simulink model "test"  (R2020a)
settings: Solver=VariableStepAuto  StartTime=0.0  StopTime=10.0  RelTol=1e-3
libraries: simulink x6, robotcorelib x2
settings Model: Creator=javier  LastModifiedBy=javier

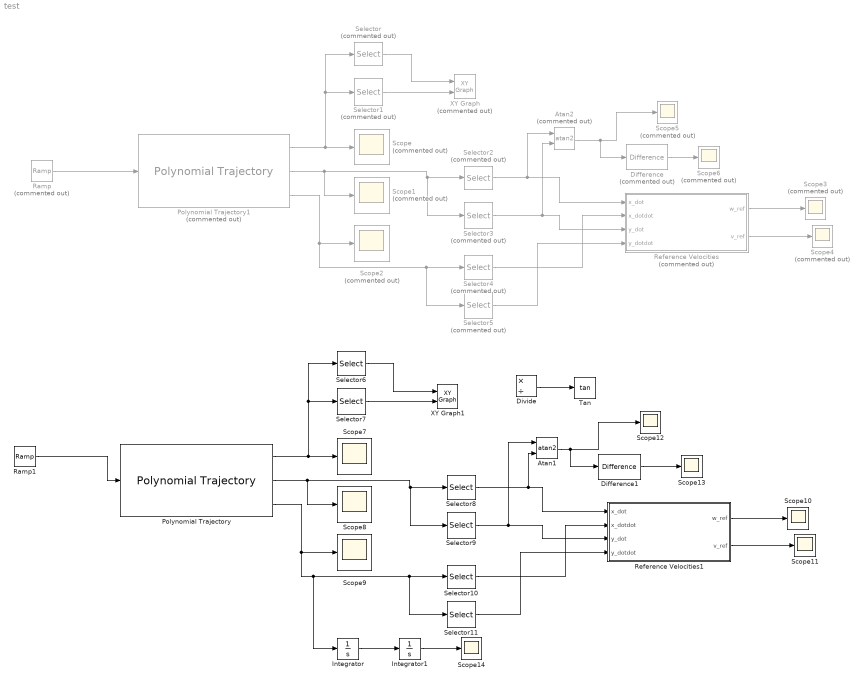
== system test ==
  Atan1 : Trigonometry  Operator=atan2  OutputSignalType=real
  Atan2 : Trigonometry  Commented=on  Operator=atan2
  Difference : simulink/Discrete/Difference  Commented=on  ICPrevInput=0.0  OutMin=[]  OutMax=[]  OutDataType=fixdt(1, 16)  OutScaling=2^-10  DoSatur=off
  Difference1 : simulink/Discrete/Difference  ICPrevInput=0  OutMin=[]  OutMax=[]  OutDataType=fixdt(1, 16)  OutScaling=2^-10  DoSatur=off
  Divide : Product  Inputs=*/
  Integrator : Integrator
  Integrator1 : Integrator
  Polynomial Trajectory : robotcorelib/Polynomial Trajectory  WaypointSource=Internal  Waypoints=[ 0, 0.5, 1, 1.5, 2, 2.5, 3; 0, 0.5, 1, 1, 1, 0.5, 0]  TimePoints=[ 0, 1, 2, 3, 4, 5, 6]  TimeInterval=[ 1, 4]  Method=Cubic Polynomial  ParameterSource=Internal  VelocityBoundaryCondition=zeros( 2, 7 )  AccelerationBoundaryCondition=zeros( 2, 4 )  SimulateUsing=Interpreted execution
      settings: SourceProductBaseCode=NV,RO,RR
  Polynomial Trajectory1 : robotcorelib/Polynomial Trajectory  Commented=on  WaypointSource=Internal  Waypoints=[ 0, 2, 1, 5, 0; -1, 3, 1, 4, 4 ]  TimePoints=[ 0, 1, 2, 3, 4 ]  TimeInterval=[ 1, 4 ]  Method=Cubic Polynomial  ParameterSource=Internal  VelocityBoundaryCondition=zeros( 2, 5 )  AccelerationBoundaryCondition=zeros( 2, 5 )  SimulateUsing=Interpreted execution
      settings: SourceProductBaseCode=NV,RO,RR
  Ramp : simulink/Sources/Ramp  Commented=on  slope=1  start=0  InitialOutput=0
  Ramp1 : simulink/Sources/Ramp  slope=1  start=0  InitialOutput=0
  Reference Velocities : Subsystem  Commented=on
  Reference Velocities1 : Subsystem
  Scope{,1..6} (7 alike) : Scope  Commented=on
  Scope{7..14} (8 alike) : Scope
  Selector : Selector  Commented=on  InputPortWidth=2  IndexOptions=Index vector (dialog)  Indices=1  OutputSizes=1
  Selector1 : Selector  Commented=on  InputPortWidth=2  IndexOptions=Index vector (dialog)  Indices=2  OutputSizes=1
  Selector10 : Selector  InputPortWidth=2  IndexOptions=Index vector (dialog)  Indices=1  OutputSizes=1
  Selector11 : Selector  InputPortWidth=2  IndexOptions=Index vector (dialog)  Indices=2  OutputSizes=1
  Selector2 : Selector  Commented=on  InputPortWidth=2  IndexOptions=Index vector (dialog)  Indices=1  OutputSizes=1
  Selector3 : Selector  Commented=on  InputPortWidth=2  IndexOptions=Index vector (dialog)  Indices=2  OutputSizes=1
  Selector4 : Selector  Commented=on  InputPortWidth=2  IndexOptions=Index vector (dialog)  Indices=1  OutputSizes=1
  Selector5 : Selector  Commented=on  InputPortWidth=2  IndexOptions=Index vector (dialog)  Indices=2  OutputSizes=1
  Selector6 : Selector  InputPortWidth=2  IndexOptions=Index vector (dialog)  Indices=1  OutputSizes=1
  Selector7 : Selector  InputPortWidth=2  IndexOptions=Index vector (dialog)  Indices=2  OutputSizes=1
  Selector8 : Selector  InputPortWidth=2  IndexOptions=Index vector (dialog)  Indices=1  OutputSizes=1
  Selector9 : Selector  InputPortWidth=2  IndexOptions=Index vector (dialog)  Indices=2  OutputSizes=1
  Tan : Trigonometry  Operator=tan
  XY Graph : simulink/Sinks/XY Graph  Commented=on  xmin=-3  xmax=5  ymin=-1  ymax=5  st=-1
  XY Graph1 : simulink/Sinks/XY Graph  xmin=-3  xmax=5  ymin=-1  ymax=5  st=-1
  wires:
  Polynomial Trajectory1/1 -> Selector1/1, Selector/1, Scope/1
  Polynomial Trajectory1/2 -> Selector3/1, Selector2/1, Scope1/1
  Selector3/1 -> Atan2/2, Reference Velocities/3(y_dot)
  Reference Velocities/1(w_ref) -> Scope3/1
  Polynomial Trajectory1/3 -> Scope2/1, Selector5/1, Selector4/1
  Selector4/1 -> Reference Velocities/2(x_dotdot)
  Atan2/1 -> Difference/1, Scope5/1
  Selector/1 -> XY Graph/1
  Selector2/1 -> Atan2/1, Reference Velocities/1(x_dot)
  Ramp/1 -> Polynomial Trajectory1/1
  Reference Velocities/2(v_ref) -> Scope4/1
  Difference/1 -> Scope6/1
  Selector5/1 -> Reference Velocities/4(y_dotdot)
  Selector1/1 -> XY Graph/2
  Selector9/1 -> Atan1/1, Reference Velocities1/3(y_dot)
  Polynomial Trajectory/2 -> Selector9/1, Selector8/1, Scope8/1
  Ramp1/1 -> Polynomial Trajectory/1
  Reference Velocities1/1(w_ref) -> Scope10/1
  Reference Velocities1/2(v_ref) -> Scope11/1
  Selector10/1 -> Reference Velocities1/2(x_dotdot)
  Selector8/1 -> Atan1/2, Reference Velocities1/1(x_dot)
  Polynomial Trajectory/1 -> Selector7/1, Selector6/1, Scope7/1
  Selector11/1 -> Reference Velocities1/4(y_dotdot)
  Polynomial Trajectory/3 -> Scope9/1, Integrator/1, Selector11/1, Selector10/1
  Atan1/1 -> Difference1/1, Scope12/1
  Selector6/1 -> XY Graph1/1
  Selector7/1 -> XY Graph1/2
  Integrator/1 -> Integrator1/1
  Integrator1/1 -> Scope14/1
  Difference1/1 -> Scope13/1
  Divide/1 -> Tan/1

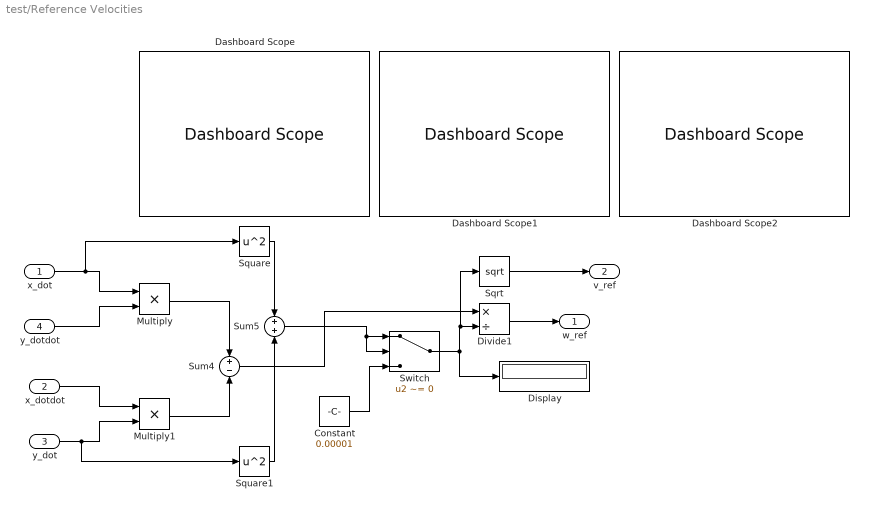
== system test/Reference Velocities ==
  x_dot : Inport
  x_dotdot : Inport  Port=2
  y_dot : Inport  Port=3
  y_dotdot : Inport  Port=4
  Constant : Constant  Value=0.00001
  Dashboard Scope : DashboardScope
  Dashboard Scope1 : DashboardScope
  Dashboard Scope2 : DashboardScope
  Display : Display
  Divide1 : Product  Inputs=*/  OutMin=[0.0000001]
  Multiply : Product
  Multiply1 : Product
  Sqrt : Sqrt  SaturateOnIntegerOverflow=on
  Square : Math  Operator=square  SignedPower=on  SaturateOnIntegerOverflow=on
  Square1 : Math  Operator=square  SignedPower=on  SaturateOnIntegerOverflow=on
  Sum4 : Sum  Inputs=+-
  Sum5 : Sum
  Switch : Switch  Criteria=u2 ~= 0
  w_ref : Outport  VectorParamsAs1DForOutWhenUnconnected=off
  v_ref : Outport  Port=2  VectorParamsAs1DForOutWhenUnconnected=off
  wires:
  x_dot/1 -> Square/1, Multiply/1
  Divide1/1 -> w_ref/1
  x_dotdot/1 -> Multiply1/1
  Square/1 -> Sum5/1
  Sum4/1 -> Divide1/1
  y_dot/1 -> Square1/1, Multiply1/2
  y_dotdot/1 -> Multiply/2
  Multiply1/1 -> Sum4/2
  Square1/1 -> Sum5/2
  Multiply/1 -> Sum4/1
  Sqrt/1 -> v_ref/1
  Constant/1 -> Switch/3
  Sum5/1 -> Switch/2, Switch/1
  Switch/1 -> Display/1, Sqrt/1, Divide1/2

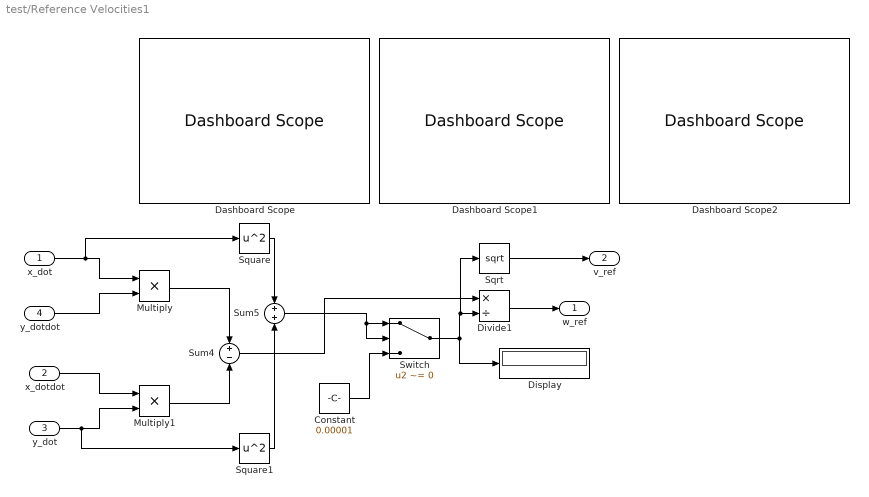
== system test/Reference Velocities1 ==
  x_dot : Inport
  x_dotdot : Inport  Port=2
  y_dot : Inport  Port=3
  y_dotdot : Inport  Port=4
  Constant : Constant  Value=0.00001
  Dashboard Scope : DashboardScope
  Dashboard Scope1 : DashboardScope
  Dashboard Scope2 : DashboardScope
  Display : Display
  Divide1 : Product  Inputs=*/  OutMin=[0.0000001]
  Multiply : Product
  Multiply1 : Product
  Sqrt : Sqrt  SaturateOnIntegerOverflow=on
  Square : Math  Operator=square  SignedPower=on  SaturateOnIntegerOverflow=on
  Square1 : Math  Operator=square  SignedPower=on  SaturateOnIntegerOverflow=on
  Sum4 : Sum  Inputs=+-
  Sum5 : Sum
  Switch : Switch  Criteria=u2 ~= 0
  w_ref : Outport  VectorParamsAs1DForOutWhenUnconnected=off
  v_ref : Outport  Port=2  VectorParamsAs1DForOutWhenUnconnected=off
  wires:
  x_dot/1 -> Square/1, Multiply/1
  Divide1/1 -> w_ref/1
  x_dotdot/1 -> Multiply1/1
  Square/1 -> Sum5/1
  Sum4/1 -> Divide1/1
  y_dot/1 -> Square1/1, Multiply1/2
  y_dotdot/1 -> Multiply/2
  Multiply1/1 -> Sum4/2
  Square1/1 -> Sum5/2
  Multiply/1 -> Sum4/1
  Sqrt/1 -> v_ref/1
  Constant/1 -> Switch/3
  Sum5/1 -> Switch/2, Switch/1
  Switch/1 -> Display/1, Sqrt/1, Divide1/2
